simulink model "opSpace_delta"  (R2018a)
settings: Solver=VariableStepAuto  StartTime=0.0  StopTime=10.0  RelTol=1e-3
values from neighbouring files (symbols this model uses):
  q0 = [0;0;0]    [HapticsSetup.m]
  x0 = interx(p(:,1),p(:,2),p(:,3),Lb,Lb,Lb,0)    [HapticsSetup.m]
  xd0 = [0;0;0]    [HapticsSetup.m]
undefined symbols (not defined in the file or in its folder): deltaJacobian, frictionMatrix, Gxmatrix, Mmatrix, Nmatrix
settings Model: Creator=klay  LastModifiedBy=augus
settings CodeAppCC: StateflowObjectComments=on

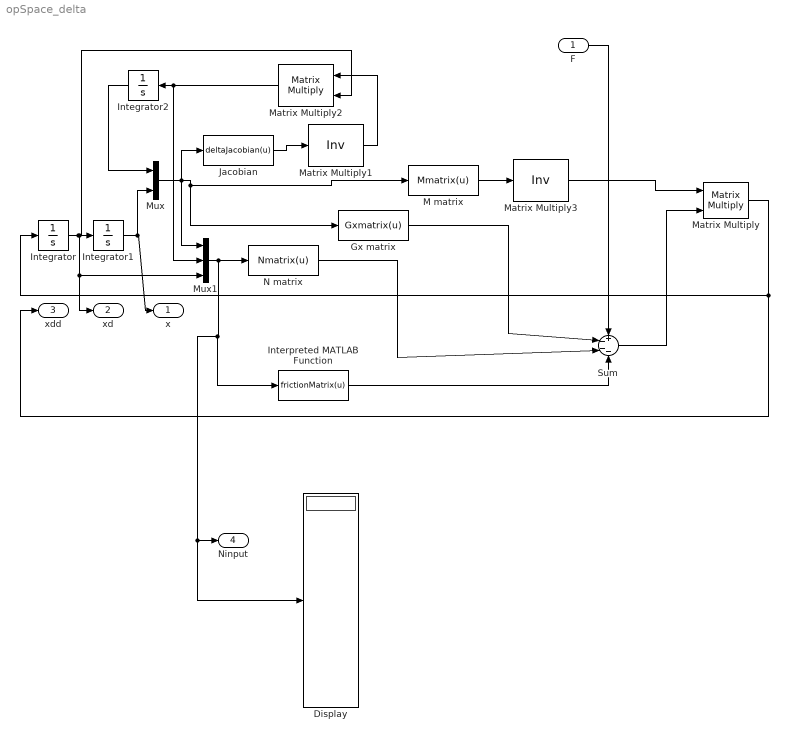
== system opSpace_delta ==
  F : Inport  PortDimensions=3
  Display : Display
  Gx matrix : MATLABFcn  MATLABFcn=Gxmatrix(u)  OutputDimensions=3  Output1D=off
  Integrator : Integrator  InitialCondition=xd0
  Integrator1 : Integrator  InitialCondition=x0
  Integrator2 : Integrator  InitialCondition=q0
  Interpreted MATLAB Function : MATLABFcn  MATLABFcn=frictionMatrix(u)  OutputDimensions=3  Output1D=off
  Jacobian : MATLABFcn  MATLABFcn=deltaJacobian(u)  Output1D=off
  M matrix : MATLABFcn  MATLABFcn=Mmatrix(u)  Output1D=off
  Matrix Multiply : Product  Multiplication=Matrix(*)
  Matrix Multiply1 : Product  Inputs=/  Multiplication=Matrix(*)
  Matrix Multiply2 : Product  Multiplication=Matrix(*)
  Matrix Multiply3 : Product  Inputs=/  Multiplication=Matrix(*)
  Mux : Mux  Inputs=2
  Mux1 : Mux  Inputs=3
  N matrix : MATLABFcn  MATLABFcn=Nmatrix(u)
  Sum : Sum  Inputs=+---
  x : Outport
  xd : Outport  Port=2
  xdd : Outport  Port=3
  "Ninput " : Outport  Port=4
  wires:
  Mux/1 -> Gx matrix/1, M matrix/1, Mux1/1, Jacobian/1
  Integrator1/1 -> Mux/2, x/1
  Jacobian/1 -> Matrix Multiply1/1
  Matrix Multiply1/1 -> Matrix Multiply2/1
  Integrator/1 -> xd/1, Mux1/3, Matrix Multiply2/2, Integrator1/1
  Integrator2/1 -> Mux/1
  Mux1/1 -> Interpreted MATLAB Function/1, "Ninput "/1, Display/1, N matrix/1
  M matrix/1 -> Matrix Multiply3/1
  Matrix Multiply3/1 -> Matrix Multiply/1
  Sum/1 -> Matrix Multiply/2
  Matrix Multiply/1 -> xdd/1, Integrator/1
  F/1 -> Sum/1
  Matrix Multiply2/1 -> Mux1/2, Integrator2/1
  Gx matrix/1 -> Sum/2
  N matrix/1 -> Sum/3
  Interpreted MATLAB Function/1 -> Sum/4
